simulink model "q1"  (R2021a)
settings: Solver=VariableStepAuto  StartTime=0.0  StopTime=8*1e-6  RelTol=1e-3
libraries: commrandsrc3 x4
settings Model: Creator=Fatiha  LastModifiedBy=Fatiha

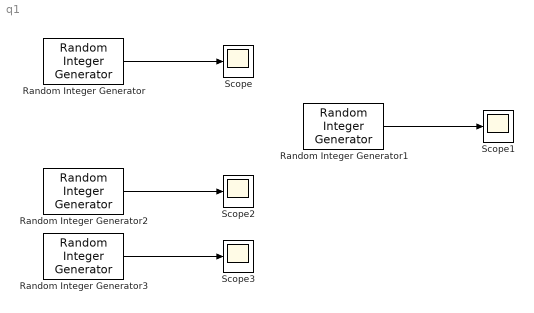
== system q1 ==
  Random Integer Generator : commrandsrc3/Random Integer Generator  SetSize=2  SeedSource=Auto  Seed=0  SampleTime=1e-6  SamplesPerFrame=1  OutputDataType=double  SimulateUsing=Interpreted execution
  Random Integer Generator1 : commrandsrc3/Random Integer Generator  SetSize=4  SeedSource=Auto  Seed=0  SampleTime=1e-6  SamplesPerFrame=1  OutputDataType=double  SimulateUsing=Interpreted execution
  Random Integer Generator2 : commrandsrc3/Random Integer Generator  SetSize=8  SeedSource=Auto  Seed=0  SampleTime=1e-6  SamplesPerFrame=1  OutputDataType=double  SimulateUsing=Interpreted execution
  Random Integer Generator3 : commrandsrc3/Random Integer Generator  SetSize=16  SeedSource=Auto  Seed=0  SampleTime=1e-6  SamplesPerFrame=1  OutputDataType=double  SimulateUsing=Interpreted execution
  Scope{,1..3} (4 alike) : Scope
  wires:
  Random Integer Generator/1 -> Scope/1
  Random Integer Generator1/1 -> Scope1/1
  Random Integer Generator2/1 -> Scope2/1
  Random Integer Generator3/1 -> Scope3/1
